simulink model "LUT_kidney_35"  (R2023b)
settings: Solver=FixedStepAuto  StartTime=0  StopTime=10.1  FixedStep=Timegap  RelTol=1e-3
model workspace (MAT data in the model file):
  T1_input = 1.34
(part 1 of 3)
settings Model: Creator=ppxmr2  LastModifiedBy=ppxmr2

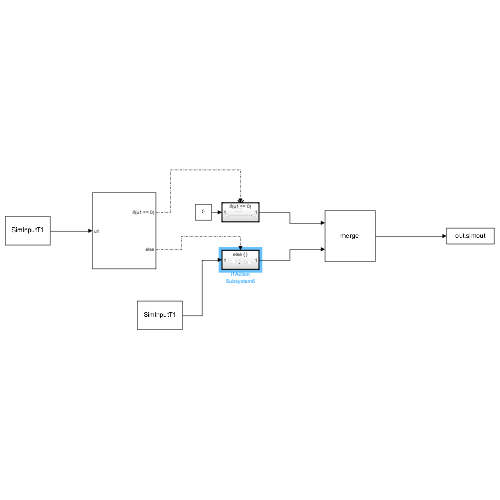
[thumbnail: Simulink's stored preview of the top-level diagram]
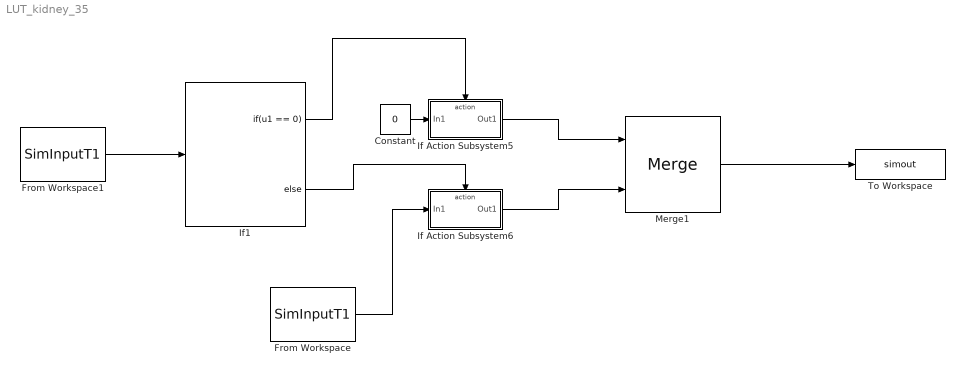
== system LUT_kidney_35 ==
  Constant : Constant  Value=0
  From Workspace : FromWorkspace  VariableName=SimInputT1  Interpolate=off  OutputAfterFinalValue=Setting to zero
  From Workspace1 : FromWorkspace  VariableName=SimInputT1  Interpolate=off  OutputAfterFinalValue=Setting to zero
  If Action Subsystem5 : Subsystem  TreatAsAtomicUnit=on
  If Action Subsystem6 : Subsystem  TreatAsAtomicUnit=on
  If1 : If  IfExpression=u1 == 0
  Merge1 : Merge
  To Workspace : ToWorkspace  VariableName=simout
  wires:
  From Workspace1/1 -> If1/1
  If1/1 -> If Action Subsystem5/Action
  If1/2 -> If Action Subsystem6/Action
  Constant/1 -> If Action Subsystem5/1(In1)
  If Action Subsystem5/1(Out1) -> Merge1/1
  If Action Subsystem6/1(Out1) -> Merge1/2
  Merge1/1 -> To Workspace/1
  From Workspace/1 -> If Action Subsystem6/1(In1)

== system LUT_kidney_35/If Action Subsystem5 ==
  In1 : Inport
  Action Port : ActionPort  ActionPortLabel=if(u1 == 0)
  Out1 : Outport
  wires:
  In1/1 -> Out1/1

== system LUT_kidney_35/If Action Subsystem6 ==
  In1 : Inport
  Action Port : ActionPort  ActionPortLabel=else
  From Workspace1 : FromWorkspace  VariableName=SimInputHR  Interpolate=off  OutputAfterFinalValue=Setting to zero
  If : If  IfExpression=u1 >= 1.495  ElseIfExpressions=u1 >= 0.995
  If Action Subsystem1 : Subsystem  TreatAsAtomicUnit=on
  If Action Subsystem2 : Subsystem  TreatAsAtomicUnit=on
  If Action Subsystem3 : Subsystem  TreatAsAtomicUnit=on
  Merge : Merge  Inputs=3
  Out1 : Outport
  wires:
  Merge/1 -> Out1/1
  From Workspace1/1 -> If/1
  If Action Subsystem1/1(Out1) -> Merge/2
  If Action Subsystem3/1(Out1) -> Merge/3
  In1/1 -> If Action Subsystem2/1(In1), If Action Subsystem1/1(In1), If Action Subsystem3/1(In1)
  If/1 -> If Action Subsystem2/Action
  If/2 -> If Action Subsystem1/Action
  If/3 -> If Action Subsystem3/Action
  If Action Subsystem2/1(Out1) -> Merge/1

== system LUT_kidney_35/If Action Subsystem6/If Action Subsystem1 ==
  In1 : Inport
  Action Port : ActionPort  ActionPortLabel=elseif(u1 >= 0.995)
  From Workspace2 : FromWorkspace  VariableName=SimInputHR  Interpolate=off  OutputAfterFinalValue=Setting to zero
  If Action Subsystem5 : Subsystem  TreatAsAtomicUnit=on
  If Action Subsystem6 : Subsystem  TreatAsAtomicUnit=on
  If Action Subsystem7 : Subsystem  TreatAsAtomicUnit=on
  If Action Subsystem8 : Subsystem  TreatAsAtomicUnit=on
  If Action Subsystem9 : Subsystem  TreatAsAtomicUnit=on
  If1 : If  IfExpression=u1 >= 1.395  ElseIfExpressions=u1 >= 1.295, u1 >= 1.195, u1 >= 1.095
  Merge1 : Merge  Inputs=5
  Out1 : Outport
  wires:
  In1/1 -> If Action Subsystem7/1(In2), If Action Subsystem8/1(In1), If Action Subsystem9/1(In1), If Action Subsystem5/1(In1), If Action Subsystem6/1(In1)
  From Workspace2/1 -> If1/1
  If Action Subsystem9/1(Out1) -> Merge1/1
  If Action Subsystem6/1(Out1) -> Merge1/5
  If Action Subsystem8/1(Out1) -> Merge1/2
  If Action Subsystem5/1(Out1) -> Merge1/4
  If1/4 -> If Action Subsystem5/Action
  If1/2 -> If Action Subsystem8/Action
  If1/3 -> If Action Subsystem7/Action
  If Action Subsystem7/1(Out2) -> Merge1/3
  If1/5 -> If Action Subsystem6/Action
  If1/1 -> If Action Subsystem9/Action
  Merge1/1 -> Out1/1

== system LUT_kidney_35/If Action Subsystem6/If Action Subsystem2 ==
  In1 : Inport
  Action Port : ActionPort  ActionPortLabel=if(u1 >= 1.495)
  From Workspace2 : FromWorkspace  VariableName=SimInputHR  Interpolate=off  OutputAfterFinalValue=Setting to zero
  If Action Subsystem5 : Subsystem  TreatAsAtomicUnit=on
  If Action Subsystem6 : Subsystem  TreatAsAtomicUnit=on
  If Action Subsystem7 : Subsystem  TreatAsAtomicUnit=on
  If Action Subsystem8 : Subsystem  TreatAsAtomicUnit=on
  If Action Subsystem9 : Subsystem  TreatAsAtomicUnit=on
  If1 : If  IfExpression=u1 >= 1.895  ElseIfExpressions=u1 >= 1.795, u1 >= 1.695, u1 >= 1.595
  Merge1 : Merge  Inputs=5
  Out1 : Outport
  wires:
  In1/1 -> If Action Subsystem9/1(In1), If Action Subsystem8/1(In1), If Action Subsystem7/1(In1), If Action Subsystem5/1(In1), If Action Subsystem6/1(In1)
  From Workspace2/1 -> If1/1
  If Action Subsystem9/1(Out1) -> Merge1/1
  If1/4 -> If Action Subsystem5/Action
  If1/2 -> If Action Subsystem8/Action
  If1/3 -> If Action Subsystem7/Action
  If1/5 -> If Action Subsystem6/Action
  If1/1 -> If Action Subsystem9/Action
  Merge1/1 -> Out1/1
  If Action Subsystem8/1(Out1) -> Merge1/2
  If Action Subsystem7/1(Out1) -> Merge1/3
  If Action Subsystem6/1(Out1) -> Merge1/5
  If Action Subsystem5/1(Out1) -> Merge1/4

== system LUT_kidney_35/If Action Subsystem6/If Action Subsystem3 ==
  In1 : Inport
  Action Port : ActionPort  ActionPortLabel=else
  From Workspace2 : FromWorkspace  VariableName=SimInputHR  Interpolate=off  OutputAfterFinalValue=Setting to zero
  If Action Subsystem5 : Subsystem  TreatAsAtomicUnit=on
  If Action Subsystem6 : Subsystem  TreatAsAtomicUnit=on
  If Action Subsystem7 : Subsystem  TreatAsAtomicUnit=on
  If Action Subsystem8 : Subsystem  TreatAsAtomicUnit=on
  If Action Subsystem9 : Subsystem  TreatAsAtomicUnit=on
  If1 : If  IfExpression=u1 >= 0.895  ElseIfExpressions=u1 >= 0.795, u1 >= 0.695, u1 >= 0595
  Merge1 : Merge  Inputs=5
  Out1 : Outport
  wires:
  In1/1 -> If Action Subsystem8/1(In1), If Action Subsystem9/1(In2), If Action Subsystem7/1(In1), If Action Subsystem5/1(In1), If Action Subsystem6/1(In1)
  From Workspace2/1 -> If1/1
  If Action Subsystem9/1(Out2) -> Merge1/1
  If Action Subsystem6/1(Out1) -> Merge1/5
  If Action Subsystem8/1(Out1) -> Merge1/2
  If Action Subsystem5/1(Out1) -> Merge1/4
  If1/4 -> If Action Subsystem5/Action
  If1/2 -> If Action Subsystem8/Action
  If1/3 -> If Action Subsystem7/Action
  If Action Subsystem7/1(Out1) -> Merge1/3
  If1/5 -> If Action Subsystem6/Action
  If1/1 -> If Action Subsystem9/Action
  Merge1/1 -> Out1/1

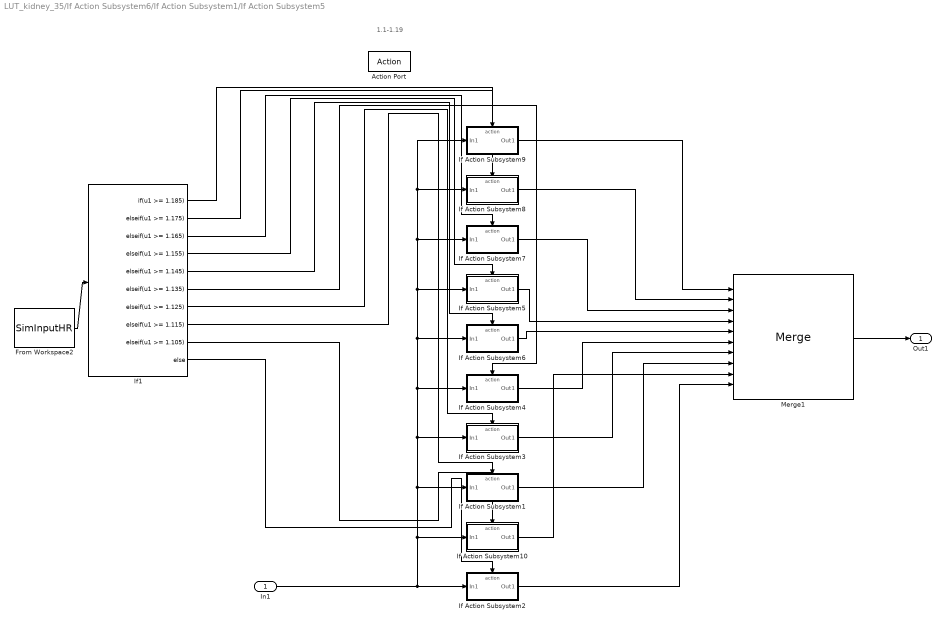
== system LUT_kidney_35/If Action Subsystem6/If Action Subsystem1/If Action Subsystem5 ==
  note: 1.1-1.19
  In1 : Inport
  Action Port : ActionPort  ActionPortLabel=elseif( u1 >= 1.095)
  From Workspace2 : FromWorkspace  VariableName=SimInputHR  Interpolate=off  OutputAfterFinalValue=Setting to zero
  If Action Subsystem1 : Subsystem  TreatAsAtomicUnit=on
  If Action Subsystem10 : Subsystem  TreatAsAtomicUnit=on
  If Action Subsystem2 : Subsystem  TreatAsAtomicUnit=on
  If Action Subsystem3 : Subsystem  TreatAsAtomicUnit=on
  If Action Subsystem4 : Subsystem  TreatAsAtomicUnit=on
  If Action Subsystem5 : Subsystem  TreatAsAtomicUnit=on
  If Action Subsystem6 : Subsystem  TreatAsAtomicUnit=on
  If Action Subsystem7 : Subsystem  TreatAsAtomicUnit=on
  If Action Subsystem8 : Subsystem  TreatAsAtomicUnit=on
  If Action Subsystem9 : Subsystem  TreatAsAtomicUnit=on
  If1 : If  IfExpression=u1 >= 1.185  ElseIfExpressions=u1 >= 1.175, u1 >= 1.165, u1 >= 1.155, u1 >= 1.145, u1 >= 1.135, u1 >= 1.125, u1 >= 1.115, u1 >= 1.105
  Merge1 : Merge  Inputs=10
  Out1 : Outport
  wires:
  If1/10 -> If Action Subsystem2/Action
  If Action Subsystem4/1(Out1) -> Merge1/6
  From Workspace2/1 -> If1/1
  If Action Subsystem6/1(Out1) -> Merge1/5
  Merge1/1 -> Out1/1
  If1/8 -> If Action Subsystem1/Action
  If Action Subsystem3/1(Out1) -> Merge1/7
  In1/1 -> If Action Subsystem1/1(In1), If Action Subsystem3/1(In1), If Action Subsystem4/1(In1), If Action Subsystem7/1(In1), If Action Subsystem8/1(In1), If Action Subsystem9/1(In1), If Action Subsystem5/1(In1), If Action Subsystem6/1(In1), If Action Subsystem10/1(In1), If Action Subsystem2/1(In1)
  If1/6 -> If Action Subsystem4/Action
  If Action Subsystem1/1(Out1) -> Merge1/8
  If1/4 -> If Action Subsystem5/Action
  If Action Subsystem8/1(Out1) -> Merge1/2
  If1/5 -> If Action Subsystem6/Action
  If Action Subsystem7/1(Out1) -> Merge1/3
  If1/3 -> If Action Subsystem7/Action
  If1/7 -> If Action Subsystem3/Action
  If Action Subsystem5/1(Out1) -> Merge1/4
  If Action Subsystem2/1(Out1) -> Merge1/10
  If1/2 -> If Action Subsystem8/Action
  If1/1 -> If Action Subsystem9/Action
  If Action Subsystem9/1(Out1) -> Merge1/1
  If1/9 -> If Action Subsystem10/Action
  If Action Subsystem10/1(Out1) -> Merge1/9

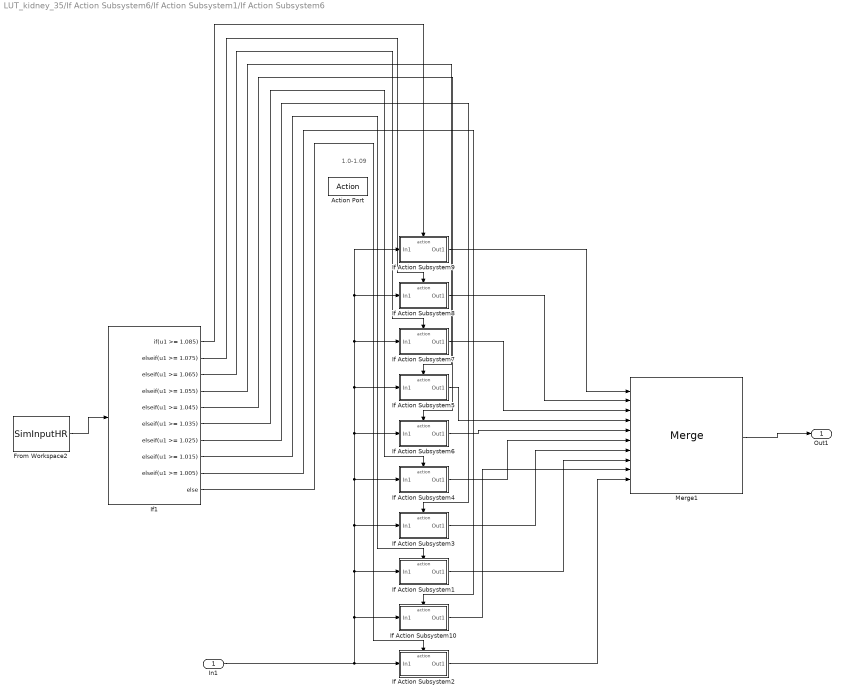
== system LUT_kidney_35/If Action Subsystem6/If Action Subsystem1/If Action Subsystem6 ==
  note: 1.0-1.09
  In1 : Inport
  Action Port : ActionPort  ActionPortLabel=else
  From Workspace2 : FromWorkspace  VariableName=SimInputHR  Interpolate=off  OutputAfterFinalValue=Setting to zero
  If Action Subsystem1 : Subsystem  TreatAsAtomicUnit=on
  If Action Subsystem10 : Subsystem  TreatAsAtomicUnit=on
  If Action Subsystem2 : Subsystem  TreatAsAtomicUnit=on
  If Action Subsystem3 : Subsystem  TreatAsAtomicUnit=on
  If Action Subsystem4 : Subsystem  TreatAsAtomicUnit=on
  If Action Subsystem5 : Subsystem  TreatAsAtomicUnit=on
  If Action Subsystem6 : Subsystem  TreatAsAtomicUnit=on
  If Action Subsystem7 : Subsystem  TreatAsAtomicUnit=on
  If Action Subsystem8 : Subsystem  TreatAsAtomicUnit=on
  If Action Subsystem9 : Subsystem  TreatAsAtomicUnit=on
  If1 : If  IfExpression=u1 >= 1.085  ElseIfExpressions=u1 >= 1.075, u1 >= 1.065, u1 >= 1.055, u1 >= 1.045, u1 >= 1.035, u1 >= 1.025, u1 >= 1.015, u1 >= 1.005
  Merge1 : Merge  Inputs=10
  Out1 : Outport
  wires:
  If1/10 -> If Action Subsystem2/Action
  If Action Subsystem4/1(Out1) -> Merge1/6
  From Workspace2/1 -> If1/1
  If Action Subsystem6/1(Out1) -> Merge1/5
  Merge1/1 -> Out1/1
  If1/8 -> If Action Subsystem1/Action
  If Action Subsystem3/1(Out1) -> Merge1/7
  In1/1 -> If Action Subsystem1/1(In1), If Action Subsystem3/1(In1), If Action Subsystem4/1(In1), If Action Subsystem7/1(In1), If Action Subsystem8/1(In1), If Action Subsystem9/1(In1), If Action Subsystem5/1(In1), If Action Subsystem6/1(In1), If Action Subsystem10/1(In1), If Action Subsystem2/1(In1)
  If1/6 -> If Action Subsystem4/Action
  If Action Subsystem1/1(Out1) -> Merge1/8
  If1/4 -> If Action Subsystem5/Action
  If Action Subsystem8/1(Out1) -> Merge1/2
  If1/5 -> If Action Subsystem6/Action
  If Action Subsystem7/1(Out1) -> Merge1/3
  If1/3 -> If Action Subsystem7/Action
  If1/7 -> If Action Subsystem3/Action
  If Action Subsystem5/1(Out1) -> Merge1/4
  If Action Subsystem2/1(Out1) -> Merge1/10
  If1/2 -> If Action Subsystem8/Action
  If1/1 -> If Action Subsystem9/Action
  If Action Subsystem9/1(Out1) -> Merge1/1
  If1/9 -> If Action Subsystem10/Action
  If Action Subsystem10/1(Out1) -> Merge1/9

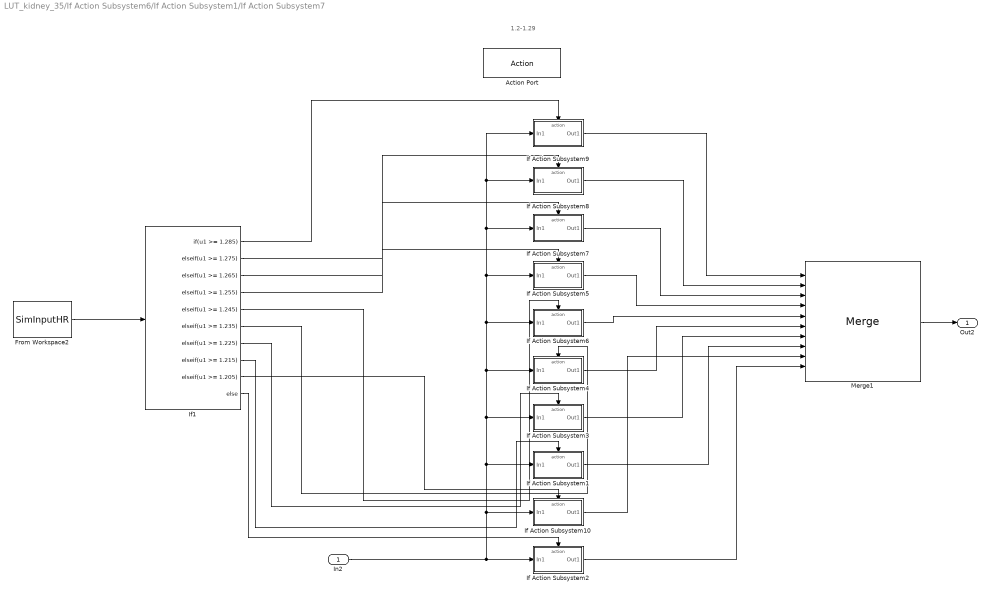
== system LUT_kidney_35/If Action Subsystem6/If Action Subsystem1/If Action Subsystem7 ==
  note: 1.2-1.29
  In2 : Inport
  Action Port : ActionPort  ActionPortLabel=elseif( u1 >= 1.195)
  From Workspace2 : FromWorkspace  VariableName=SimInputHR  Interpolate=off  OutputAfterFinalValue=Setting to zero
  If Action Subsystem1 : Subsystem  TreatAsAtomicUnit=on
  If Action Subsystem10 : Subsystem  TreatAsAtomicUnit=on
  If Action Subsystem2 : Subsystem  TreatAsAtomicUnit=on
  If Action Subsystem3 : Subsystem  TreatAsAtomicUnit=on
  If Action Subsystem4 : Subsystem  TreatAsAtomicUnit=on
  If Action Subsystem5 : Subsystem  TreatAsAtomicUnit=on
  If Action Subsystem6 : Subsystem  TreatAsAtomicUnit=on
  If Action Subsystem7 : Subsystem  TreatAsAtomicUnit=on
  If Action Subsystem8 : Subsystem  TreatAsAtomicUnit=on
  If Action Subsystem9 : Subsystem  TreatAsAtomicUnit=on
  If1 : If  IfExpression=u1 >= 1.285  ElseIfExpressions=u1 >= 1.275, u1 >= 1.265, u1 >= 1.255, u1 >= 1.245, u1 >= 1.235, u1 >= 1.225, u1 >= 1.215, u1 >= 1.205
  Merge1 : Merge  Inputs=10
  Out2 : Outport
  wires:
  If1/10 -> If Action Subsystem2/Action
  If Action Subsystem4/1(Out1) -> Merge1/6
  From Workspace2/1 -> If1/1
  If Action Subsystem6/1(Out1) -> Merge1/5
  Merge1/1 -> Out2/1
  If1/8 -> If Action Subsystem1/Action
  If Action Subsystem3/1(Out1) -> Merge1/7
  In2/1 -> If Action Subsystem1/1(In1), If Action Subsystem3/1(In1), If Action Subsystem4/1(In1), If Action Subsystem7/1(In1), If Action Subsystem8/1(In1), If Action Subsystem9/1(In1), If Action Subsystem5/1(In1), If Action Subsystem6/1(In1), If Action Subsystem10/1(In1), If Action Subsystem2/1(In1)
  If1/6 -> If Action Subsystem4/Action
  If Action Subsystem1/1(Out1) -> Merge1/8
  If1/4 -> If Action Subsystem5/Action
  If Action Subsystem8/1(Out1) -> Merge1/2
  If1/5 -> If Action Subsystem6/Action
  If Action Subsystem7/1(Out1) -> Merge1/3
  If1/3 -> If Action Subsystem7/Action
  If1/7 -> If Action Subsystem3/Action
  If Action Subsystem5/1(Out1) -> Merge1/4
  If Action Subsystem2/1(Out1) -> Merge1/10
  If1/2 -> If Action Subsystem8/Action
  If1/1 -> If Action Subsystem9/Action
  If Action Subsystem9/1(Out1) -> Merge1/1
  If Action Subsystem10/1(Out1) -> Merge1/9
  If1/9 -> If Action Subsystem10/Action

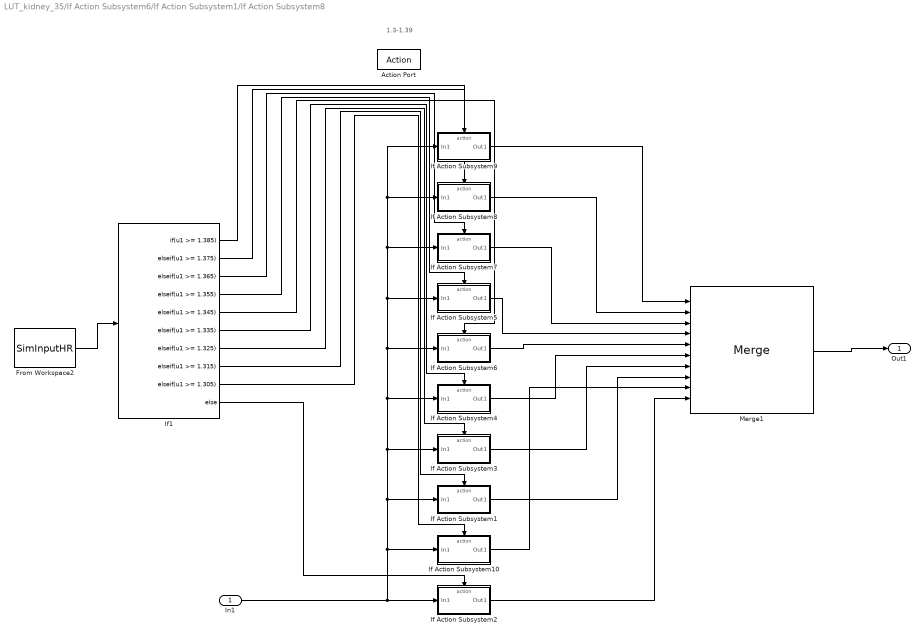
== system LUT_kidney_35/If Action Subsystem6/If Action Subsystem1/If Action Subsystem8 ==
  note: 1.3-1.39
  In1 : Inport
  Action Port : ActionPort  ActionPortLabel=elseif(u1 >= 1.295)
  From Workspace2 : FromWorkspace  VariableName=SimInputHR  Interpolate=off  OutputAfterFinalValue=Setting to zero
  If Action Subsystem1 : Subsystem  TreatAsAtomicUnit=on
  If Action Subsystem10 : Subsystem  TreatAsAtomicUnit=on
  If Action Subsystem2 : Subsystem  TreatAsAtomicUnit=on
  If Action Subsystem3 : Subsystem  TreatAsAtomicUnit=on
  If Action Subsystem4 : Subsystem  TreatAsAtomicUnit=on
  If Action Subsystem5 : Subsystem  TreatAsAtomicUnit=on
  If Action Subsystem6 : Subsystem  TreatAsAtomicUnit=on
  If Action Subsystem7 : Subsystem  TreatAsAtomicUnit=on
  If Action Subsystem8 : Subsystem  TreatAsAtomicUnit=on
  If Action Subsystem9 : Subsystem  TreatAsAtomicUnit=on
  If1 : If  IfExpression=u1 >= 1.385  ElseIfExpressions=u1 >= 1.375, u1 >= 1.365, u1 >= 1.355, u1 >= 1.345, u1 >= 1.335, u1 >= 1.325, u1 >= 1.315, u1 >= 1.305
  Merge1 : Merge  Inputs=10
  Out1 : Outport
  wires:
  If1/10 -> If Action Subsystem2/Action
  If Action Subsystem4/1(Out1) -> Merge1/6
  From Workspace2/1 -> If1/1
  If Action Subsystem6/1(Out1) -> Merge1/5
  Merge1/1 -> Out1/1
  If1/8 -> If Action Subsystem1/Action
  If Action Subsystem3/1(Out1) -> Merge1/7
  In1/1 -> If Action Subsystem1/1(In1), If Action Subsystem3/1(In1), If Action Subsystem4/1(In1), If Action Subsystem7/1(In1), If Action Subsystem8/1(In1), If Action Subsystem9/1(In1), If Action Subsystem5/1(In1), If Action Subsystem6/1(In1), If Action Subsystem10/1(In1), If Action Subsystem2/1(In1)
  If1/6 -> If Action Subsystem4/Action
  If Action Subsystem1/1(Out1) -> Merge1/8
  If1/4 -> If Action Subsystem5/Action
  If Action Subsystem8/1(Out1) -> Merge1/2
  If1/5 -> If Action Subsystem6/Action
  If Action Subsystem7/1(Out1) -> Merge1/3
  If1/3 -> If Action Subsystem7/Action
  If1/7 -> If Action Subsystem3/Action
  If Action Subsystem5/1(Out1) -> Merge1/4
  If Action Subsystem2/1(Out1) -> Merge1/10
  If1/2 -> If Action Subsystem8/Action
  If1/1 -> If Action Subsystem9/Action
  If Action Subsystem9/1(Out1) -> Merge1/1
  If1/9 -> If Action Subsystem10/Action
  If Action Subsystem10/1(Out1) -> Merge1/9

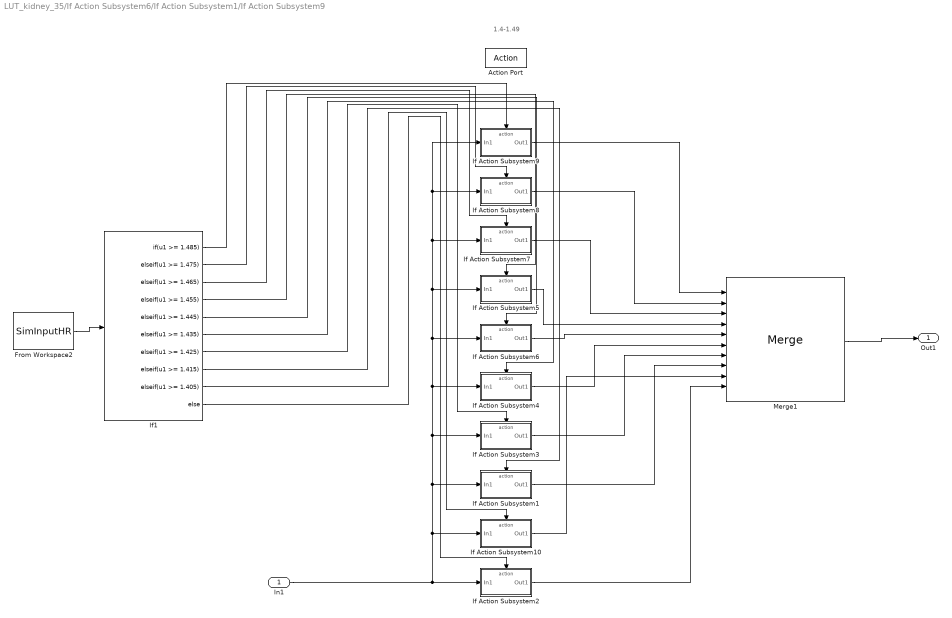
== system LUT_kidney_35/If Action Subsystem6/If Action Subsystem1/If Action Subsystem9 ==
  note: 1.4-1.49
  In1 : Inport
  Action Port : ActionPort  ActionPortLabel=if(u1 >= 1.395)
  From Workspace2 : FromWorkspace  VariableName=SimInputHR  Interpolate=off  OutputAfterFinalValue=Setting to zero
  If Action Subsystem1 : Subsystem  TreatAsAtomicUnit=on
  If Action Subsystem10 : Subsystem  TreatAsAtomicUnit=on
  If Action Subsystem2 : Subsystem  TreatAsAtomicUnit=on
  If Action Subsystem3 : Subsystem  TreatAsAtomicUnit=on
  If Action Subsystem4 : Subsystem  TreatAsAtomicUnit=on
  If Action Subsystem5 : Subsystem  TreatAsAtomicUnit=on
  If Action Subsystem6 : Subsystem  TreatAsAtomicUnit=on
  If Action Subsystem7 : Subsystem  TreatAsAtomicUnit=on
  If Action Subsystem8 : Subsystem  TreatAsAtomicUnit=on
  If Action Subsystem9 : Subsystem  TreatAsAtomicUnit=on
  If1 : If  IfExpression=u1 >= 1.485  ElseIfExpressions=u1 >= 1.475, u1 >= 1.465, u1 >= 1.455, u1 >= 1.445, u1 >= 1.435, u1 >= 1.425, u1 >= 1.415, u1 >= 1.405
  Merge1 : Merge  Inputs=10
  Out1 : Outport
  wires:
  If1/10 -> If Action Subsystem2/Action
  If Action Subsystem4/1(Out1) -> Merge1/6
  From Workspace2/1 -> If1/1
  If Action Subsystem6/1(Out1) -> Merge1/5
  Merge1/1 -> Out1/1
  If1/8 -> If Action Subsystem1/Action
  If Action Subsystem3/1(Out1) -> Merge1/7
  In1/1 -> If Action Subsystem10/1(In1), If Action Subsystem1/1(In1), If Action Subsystem3/1(In1), If Action Subsystem4/1(In1), If Action Subsystem7/1(In1), If Action Subsystem8/1(In1), If Action Subsystem9/1(In1), If Action Subsystem5/1(In1), If Action Subsystem6/1(In1), If Action Subsystem2/1(In1)
  If1/6 -> If Action Subsystem4/Action
  If Action Subsystem1/1(Out1) -> Merge1/8
  If1/4 -> If Action Subsystem5/Action
  If Action Subsystem8/1(Out1) -> Merge1/2
  If1/5 -> If Action Subsystem6/Action
  If Action Subsystem7/1(Out1) -> Merge1/3
  If1/3 -> If Action Subsystem7/Action
  If1/7 -> If Action Subsystem3/Action
  If Action Subsystem5/1(Out1) -> Merge1/4
  If Action Subsystem2/1(Out1) -> Merge1/10
  If1/2 -> If Action Subsystem8/Action
  If1/1 -> If Action Subsystem9/Action
  If Action Subsystem9/1(Out1) -> Merge1/1
  If1/9 -> If Action Subsystem10/Action
  If Action Subsystem10/1(Out1) -> Merge1/9

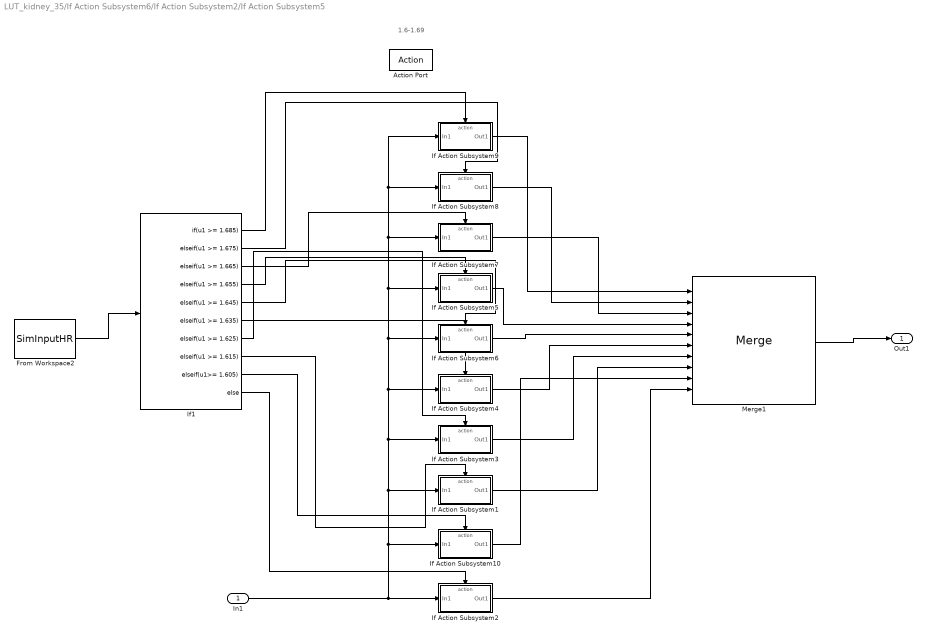
== system LUT_kidney_35/If Action Subsystem6/If Action Subsystem2/If Action Subsystem5 ==
  note: 1.6-1.69
  In1 : Inport
  Action Port : ActionPort  ActionPortLabel=elseif( u1 >= 1.595)
  From Workspace2 : FromWorkspace  VariableName=SimInputHR  Interpolate=off  OutputAfterFinalValue=Setting to zero
  If Action Subsystem1 : Subsystem  TreatAsAtomicUnit=on
  If Action Subsystem10 : Subsystem  TreatAsAtomicUnit=on
  If Action Subsystem2 : Subsystem  TreatAsAtomicUnit=on
  If Action Subsystem3 : Subsystem  TreatAsAtomicUnit=on
  If Action Subsystem4 : Subsystem  TreatAsAtomicUnit=on
  If Action Subsystem5 : Subsystem  TreatAsAtomicUnit=on
  If Action Subsystem6 : Subsystem  TreatAsAtomicUnit=on
  If Action Subsystem7 : Subsystem  TreatAsAtomicUnit=on
  If Action Subsystem8 : Subsystem  TreatAsAtomicUnit=on
  If Action Subsystem9 : Subsystem  TreatAsAtomicUnit=on
  If1 : If  IfExpression=u1 >= 1.685  ElseIfExpressions=u1 >= 1.675, u1 >= 1.665, u1 >= 1.655, u1 >= 1.645, u1 >= 1.635, u1 >= 1.625, u1 >= 1.615, u1>= 1.605
  Merge1 : Merge  Inputs=10
  Out1 : Outport
  wires:
  If1/2 -> If Action Subsystem8/Action
  If Action Subsystem5/1(Out1) -> Merge1/4
  If1/3 -> If Action Subsystem7/Action
  If Action Subsystem9/1(Out1) -> Merge1/1
  If1/7 -> If Action Subsystem3/Action
  If1/5 -> If Action Subsystem6/Action
  If1/1 -> If Action Subsystem9/Action
  If Action Subsystem4/1(Out1) -> Merge1/6
  If1/10 -> If Action Subsystem2/Action
  If Action Subsystem8/1(Out1) -> Merge1/2
  If1/4 -> If Action Subsystem5/Action
  In1/1 -> If Action Subsystem10/1(In1), If Action Subsystem1/1(In1), If Action Subsystem3/1(In1), If Action Subsystem4/1(In1), If Action Subsystem7/1(In1), If Action Subsystem8/1(In1), If Action Subsystem9/1(In1), If Action Subsystem5/1(In1), If Action Subsystem6/1(In1), If Action Subsystem2/1(In1)
  If Action Subsystem1/1(Out1) -> Merge1/8
  If Action Subsystem2/1(Out1) -> Merge1/10
  If1/8 -> If Action Subsystem1/Action
  If Action Subsystem3/1(Out1) -> Merge1/7
  If1/6 -> If Action Subsystem4/Action
  From Workspace2/1 -> If1/1
  Merge1/1 -> Out1/1
  If Action Subsystem6/1(Out1) -> Merge1/5
  If Action Subsystem7/1(Out1) -> Merge1/3
  If1/9 -> If Action Subsystem10/Action
  If Action Subsystem10/1(Out1) -> Merge1/9

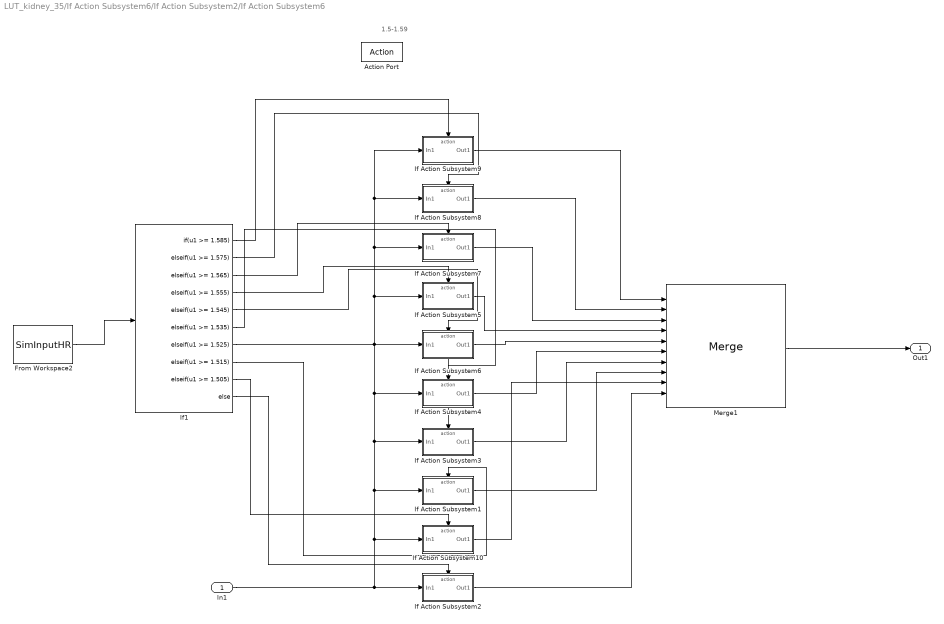
== system LUT_kidney_35/If Action Subsystem6/If Action Subsystem2/If Action Subsystem6 ==
  note: 1.5-1.59
  In1 : Inport
  Action Port : ActionPort  ActionPortLabel=else
  From Workspace2 : FromWorkspace  VariableName=SimInputHR  Interpolate=off  OutputAfterFinalValue=Setting to zero
  If Action Subsystem1 : Subsystem  TreatAsAtomicUnit=on
  If Action Subsystem10 : Subsystem  TreatAsAtomicUnit=on
  If Action Subsystem2 : Subsystem  TreatAsAtomicUnit=on
  If Action Subsystem3 : Subsystem  TreatAsAtomicUnit=on
  If Action Subsystem4 : Subsystem  TreatAsAtomicUnit=on
  If Action Subsystem5 : Subsystem  TreatAsAtomicUnit=on
  If Action Subsystem6 : Subsystem  TreatAsAtomicUnit=on
  If Action Subsystem7 : Subsystem  TreatAsAtomicUnit=on
  If Action Subsystem8 : Subsystem  TreatAsAtomicUnit=on
  If Action Subsystem9 : Subsystem  TreatAsAtomicUnit=on
  If1 : If  IfExpression=u1 >= 1.585  ElseIfExpressions=u1 >= 1.575, u1 >= 1.565, u1 >= 1.555, u1 >= 1.545, u1 >= 1.535, u1 >= 1.525, u1 >= 1.515, u1 >= 1.505
  Merge1 : Merge  Inputs=10
  Out1 : Outport
  wires:
  If1/2 -> If Action Subsystem8/Action
  If Action Subsystem5/1(Out1) -> Merge1/4
  If1/3 -> If Action Subsystem7/Action
  If Action Subsystem9/1(Out1) -> Merge1/1
  If1/7 -> If Action Subsystem3/Action
  If1/5 -> If Action Subsystem6/Action
  If1/1 -> If Action Subsystem9/Action
  If Action Subsystem4/1(Out1) -> Merge1/6
  If1/10 -> If Action Subsystem2/Action
  If Action Subsystem8/1(Out1) -> Merge1/2
  If1/4 -> If Action Subsystem5/Action
  In1/1 -> If Action Subsystem10/1(In1), If Action Subsystem1/1(In1), If Action Subsystem3/1(In1), If Action Subsystem4/1(In1), If Action Subsystem7/1(In1), If Action Subsystem8/1(In1), If Action Subsystem9/1(In1), If Action Subsystem5/1(In1), If Action Subsystem6/1(In1), If Action Subsystem2/1(In1)
  If Action Subsystem1/1(Out1) -> Merge1/8
  If Action Subsystem2/1(Out1) -> Merge1/10
  If1/8 -> If Action Subsystem1/Action
  If Action Subsystem3/1(Out1) -> Merge1/7
  If1/6 -> If Action Subsystem4/Action
  From Workspace2/1 -> If1/1
  Merge1/1 -> Out1/1
  If Action Subsystem6/1(Out1) -> Merge1/5
  If Action Subsystem7/1(Out1) -> Merge1/3
  If1/9 -> If Action Subsystem10/Action
  If Action Subsystem10/1(Out1) -> Merge1/9

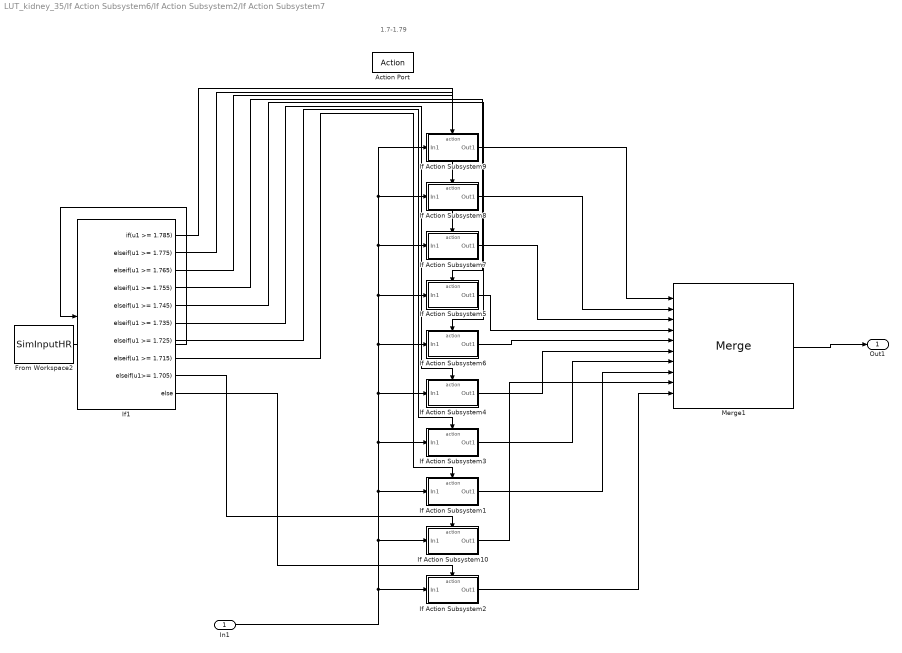
== system LUT_kidney_35/If Action Subsystem6/If Action Subsystem2/If Action Subsystem7 ==
  note: 1.7-1.79
  In1 : Inport
  Action Port : ActionPort  ActionPortLabel=elseif( u1 >= 1.695)
  From Workspace2 : FromWorkspace  VariableName=SimInputHR  Interpolate=off  OutputAfterFinalValue=Setting to zero
  If Action Subsystem1 : Subsystem  TreatAsAtomicUnit=on
  If Action Subsystem10 : Subsystem  TreatAsAtomicUnit=on
  If Action Subsystem2 : Subsystem  TreatAsAtomicUnit=on
  If Action Subsystem3 : Subsystem  TreatAsAtomicUnit=on
  If Action Subsystem4 : Subsystem  TreatAsAtomicUnit=on
  If Action Subsystem5 : Subsystem  TreatAsAtomicUnit=on
  If Action Subsystem6 : Subsystem  TreatAsAtomicUnit=on
  If Action Subsystem7 : Subsystem  TreatAsAtomicUnit=on
  If Action Subsystem8 : Subsystem  TreatAsAtomicUnit=on
  If Action Subsystem9 : Subsystem  TreatAsAtomicUnit=on
  If1 : If  IfExpression=u1 >= 1.785  ElseIfExpressions=u1 >= 1.775, u1 >= 1.765, u1 >= 1.755, u1 >= 1.745, u1 >= 1.735, u1 >= 1.725, u1 >= 1.715, u1>= 1.705
  Merge1 : Merge  Inputs=10
  Out1 : Outport
  wires:
  If1/2 -> If Action Subsystem8/Action
  If Action Subsystem5/1(Out1) -> Merge1/4
  If1/3 -> If Action Subsystem7/Action
  If Action Subsystem9/1(Out1) -> Merge1/1
  If1/7 -> If Action Subsystem3/Action
  If1/5 -> If Action Subsystem6/Action
  If1/1 -> If Action Subsystem9/Action
  If Action Subsystem4/1(Out1) -> Merge1/6
  If1/10 -> If Action Subsystem2/Action
  If Action Subsystem8/1(Out1) -> Merge1/2
  If1/4 -> If Action Subsystem5/Action
  In1/1 -> If Action Subsystem10/1(In1), If Action Subsystem1/1(In1), If Action Subsystem3/1(In1), If Action Subsystem4/1(In1), If Action Subsystem7/1(In1), If Action Subsystem8/1(In1), If Action Subsystem9/1(In1), If Action Subsystem5/1(In1), If Action Subsystem6/1(In1), If Action Subsystem2/1(In1)
  If Action Subsystem1/1(Out1) -> Merge1/8
  If Action Subsystem2/1(Out1) -> Merge1/10
  If1/8 -> If Action Subsystem1/Action
  If Action Subsystem3/1(Out1) -> Merge1/7
  If1/6 -> If Action Subsystem4/Action
  From Workspace2/1 -> If1/1
  Merge1/1 -> Out1/1
  If Action Subsystem6/1(Out1) -> Merge1/5
  If Action Subsystem7/1(Out1) -> Merge1/3
  If Action Subsystem10/1(Out1) -> Merge1/9
  If1/9 -> If Action Subsystem10/Action

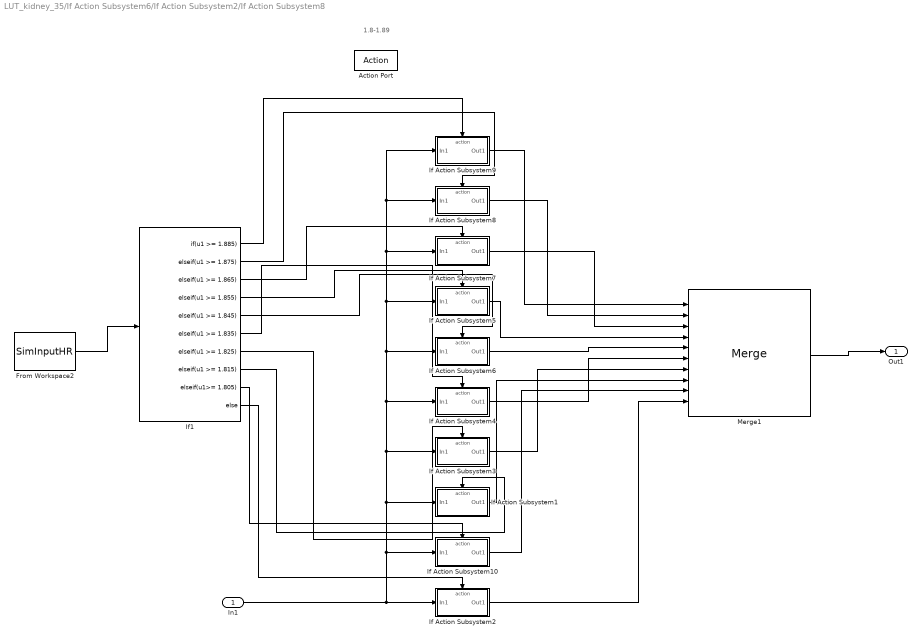
== system LUT_kidney_35/If Action Subsystem6/If Action Subsystem2/If Action Subsystem8 ==
  note: 1.8-1.89
  In1 : Inport
  Action Port : ActionPort  ActionPortLabel=elseif(u1 >= 1.795)
  From Workspace2 : FromWorkspace  VariableName=SimInputHR  Interpolate=off  OutputAfterFinalValue=Setting to zero
  If Action Subsystem1 : Subsystem  TreatAsAtomicUnit=on
  If Action Subsystem10 : Subsystem  TreatAsAtomicUnit=on
  If Action Subsystem2 : Subsystem  TreatAsAtomicUnit=on
  If Action Subsystem3 : Subsystem  TreatAsAtomicUnit=on
  If Action Subsystem4 : Subsystem  TreatAsAtomicUnit=on
  If Action Subsystem5 : Subsystem  TreatAsAtomicUnit=on
  If Action Subsystem6 : Subsystem  TreatAsAtomicUnit=on
  If Action Subsystem7 : Subsystem  TreatAsAtomicUnit=on
  If Action Subsystem8 : Subsystem  TreatAsAtomicUnit=on
  If Action Subsystem9 : Subsystem  TreatAsAtomicUnit=on
  If1 : If  IfExpression=u1 >= 1.885  ElseIfExpressions=u1 >= 1.875, u1 >= 1.865, u1 >= 1.855, u1 >= 1.845, u1 >= 1.835, u1 >= 1.825, u1 >= 1.815, u1>= 1.805
  Merge1 : Merge  Inputs=10
  Out1 : Outport
  wires:
  If1/2 -> If Action Subsystem8/Action
  If Action Subsystem5/1(Out1) -> Merge1/4
  If1/3 -> If Action Subsystem7/Action
  If Action Subsystem9/1(Out1) -> Merge1/1
  If1/7 -> If Action Subsystem3/Action
  If1/5 -> If Action Subsystem6/Action
  If1/1 -> If Action Subsystem9/Action
  If Action Subsystem4/1(Out1) -> Merge1/6
  If1/10 -> If Action Subsystem2/Action
  If Action Subsystem8/1(Out1) -> Merge1/2
  If1/4 -> If Action Subsystem5/Action
  In1/1 -> If Action Subsystem10/1(In1), If Action Subsystem1/1(In1), If Action Subsystem3/1(In1), If Action Subsystem4/1(In1), If Action Subsystem7/1(In1), If Action Subsystem8/1(In1), If Action Subsystem9/1(In1), If Action Subsystem5/1(In1), If Action Subsystem6/1(In1), If Action Subsystem2/1(In1)
  If Action Subsystem1/1(Out1) -> Merge1/8
  If Action Subsystem2/1(Out1) -> Merge1/10
  If1/8 -> If Action Subsystem1/Action
  If Action Subsystem3/1(Out1) -> Merge1/7
  If1/6 -> If Action Subsystem4/Action
  From Workspace2/1 -> If1/1
  Merge1/1 -> Out1/1
  If Action Subsystem6/1(Out1) -> Merge1/5
  If Action Subsystem7/1(Out1) -> Merge1/3
  If1/9 -> If Action Subsystem10/Action
  If Action Subsystem10/1(Out1) -> Merge1/9

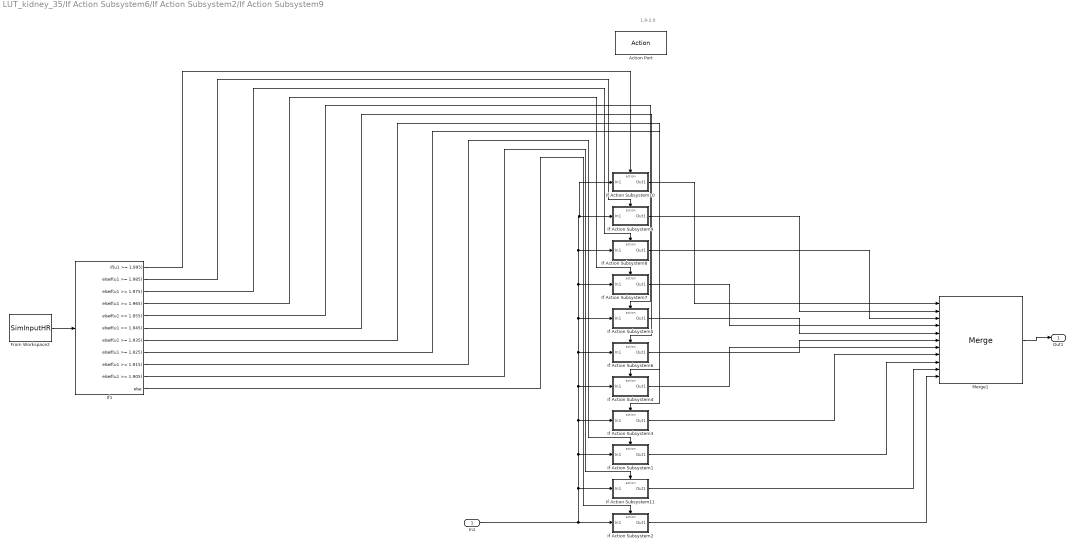
== system LUT_kidney_35/If Action Subsystem6/If Action Subsystem2/If Action Subsystem9 ==
  note: 1.9-2.0
  In1 : Inport
  Action Port : ActionPort  ActionPortLabel=if(u1 >= 1.895)
  From Workspace2 : FromWorkspace  VariableName=SimInputHR  Interpolate=off  OutputAfterFinalValue=Setting to zero
  If Action Subsystem1 : Subsystem  TreatAsAtomicUnit=on
  If Action Subsystem10 : Subsystem  TreatAsAtomicUnit=on
  If Action Subsystem11 : Subsystem  TreatAsAtomicUnit=on
  If Action Subsystem2 : Subsystem  TreatAsAtomicUnit=on
  If Action Subsystem3 : Subsystem  TreatAsAtomicUnit=on
  If Action Subsystem4 : Subsystem  TreatAsAtomicUnit=on
  If Action Subsystem5 : Subsystem  TreatAsAtomicUnit=on
  If Action Subsystem6 : Subsystem  TreatAsAtomicUnit=on
  If Action Subsystem7 : Subsystem  TreatAsAtomicUnit=on
  If Action Subsystem8 : Subsystem  TreatAsAtomicUnit=on
  If Action Subsystem9 : Subsystem  TreatAsAtomicUnit=on
  If1 : If  IfExpression=u1 >= 1.995  ElseIfExpressions=u1 >= 1.985, u1 >= 1.975, u1 >= 1.965, u1 >= 1.955, u1 >= 1.945, u1 >= 1.935, u1 >= 1.925, u1 >= 1.915, u1 >= 1.905
  Merge1 : Merge  Inputs=11
  Out1 : Outport
  wires:
  Merge1/1 -> Out1/1
  From Workspace2/1 -> If1/1
  If1/2 -> If Action Subsystem9/Action
  If1/3 -> If Action Subsystem8/Action
  If1/4 -> If Action Subsystem7/Action
  If1/5 -> If Action Subsystem5/Action
  If1/6 -> If Action Subsystem6/Action
  If1/7 -> If Action Subsystem4/Action
  If1/8 -> If Action Subsystem3/Action
  If1/9 -> If Action Subsystem1/Action
  If1/11 -> If Action Subsystem2/Action
  If Action Subsystem9/1(Out1) -> Merge1/2
  If Action Subsystem8/1(Out1) -> Merge1/3
  If Action Subsystem7/1(Out1) -> Merge1/4
  If Action Subsystem5/1(Out1) -> Merge1/5
  If Action Subsystem6/1(Out1) -> Merge1/6
  If Action Subsystem4/1(Out1) -> Merge1/7
  If Action Subsystem3/1(Out1) -> Merge1/8
  If Action Subsystem2/1(Out1) -> Merge1/11
  If Action Subsystem1/1(Out1) -> Merge1/9
  In1/1 -> If Action Subsystem1/1(In1), If Action Subsystem3/1(In1), If Action Subsystem4/1(In1), If Action Subsystem7/1(In1), If Action Subsystem8/1(In1), If Action Subsystem10/1(In1), If Action Subsystem9/1(In1), If Action Subsystem5/1(In1), If Action Subsystem6/1(In1), If Action Subsystem11/1(In1), If Action Subsystem2/1(In1)
  If1/1 -> If Action Subsystem10/Action
  If Action Subsystem10/1(Out1) -> Merge1/1
  If1/10 -> If Action Subsystem11/Action
  If Action Subsystem11/1(Out1) -> Merge1/10

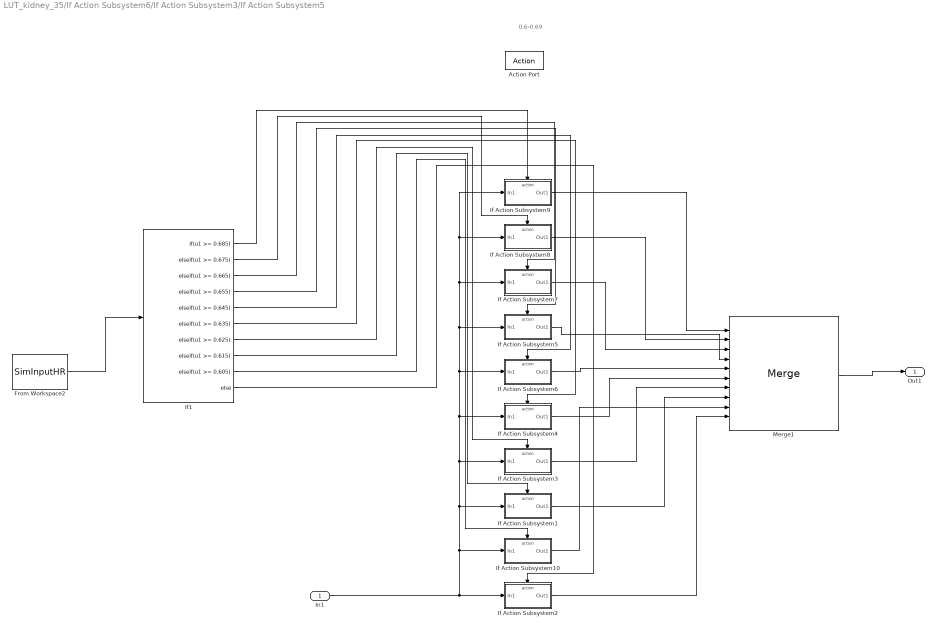
== system LUT_kidney_35/If Action Subsystem6/If Action Subsystem3/If Action Subsystem5 ==
  note: 0.6-0.69
  In1 : Inport
  Action Port : ActionPort  ActionPortLabel=elseif( u1 >= 0595)
  From Workspace2 : FromWorkspace  VariableName=SimInputHR  Interpolate=off  OutputAfterFinalValue=Setting to zero
  If Action Subsystem1 : Subsystem  TreatAsAtomicUnit=on
  If Action Subsystem10 : Subsystem  TreatAsAtomicUnit=on
  If Action Subsystem2 : Subsystem  TreatAsAtomicUnit=on
  If Action Subsystem3 : Subsystem  TreatAsAtomicUnit=on
  If Action Subsystem4 : Subsystem  TreatAsAtomicUnit=on
  If Action Subsystem5 : Subsystem  TreatAsAtomicUnit=on
  If Action Subsystem6 : Subsystem  TreatAsAtomicUnit=on
  If Action Subsystem7 : Subsystem  TreatAsAtomicUnit=on
  If Action Subsystem8 : Subsystem  TreatAsAtomicUnit=on
  If Action Subsystem9 : Subsystem  TreatAsAtomicUnit=on
  If1 : If  IfExpression=u1 >= 0.685  ElseIfExpressions=u1 >= 0.675, u1 >= 0.665, u1 >= 0.655, u1 >= 0.645, u1 >= 0.635, u1 >= 0.625, u1 >= 0.615, u1 >= 0.605
  Merge1 : Merge  Inputs=10
  Out1 : Outport
  wires:
  If1/10 -> If Action Subsystem2/Action
  If Action Subsystem4/1(Out1) -> Merge1/6
  From Workspace2/1 -> If1/1
  If Action Subsystem6/1(Out1) -> Merge1/5
  Merge1/1 -> Out1/1
  If1/8 -> If Action Subsystem1/Action
  If Action Subsystem3/1(Out1) -> Merge1/7
  In1/1 -> If Action Subsystem1/1(In1), If Action Subsystem3/1(In1), If Action Subsystem4/1(In1), If Action Subsystem7/1(In1), If Action Subsystem8/1(In1), If Action Subsystem9/1(In1), If Action Subsystem5/1(In1), If Action Subsystem6/1(In1), If Action Subsystem10/1(In1), If Action Subsystem2/1(In1)
  If1/6 -> If Action Subsystem4/Action
  If Action Subsystem1/1(Out1) -> Merge1/8
  If1/4 -> If Action Subsystem5/Action
  If Action Subsystem8/1(Out1) -> Merge1/2
  If1/5 -> If Action Subsystem6/Action
  If Action Subsystem7/1(Out1) -> Merge1/3
  If1/3 -> If Action Subsystem7/Action
  If1/7 -> If Action Subsystem3/Action
  If Action Subsystem5/1(Out1) -> Merge1/4
  If Action Subsystem2/1(Out1) -> Merge1/10
  If1/2 -> If Action Subsystem8/Action
  If1/1 -> If Action Subsystem9/Action
  If Action Subsystem9/1(Out1) -> Merge1/1
  If Action Subsystem10/1(Out1) -> Merge1/9
  If1/9 -> If Action Subsystem10/Action

== system LUT_kidney_35/If Action Subsystem6/If Action Subsystem3/If Action Subsystem6 ==
  note: 0.5-0.59
  In1 : Inport
  Action Port : ActionPort  ActionPortLabel=else
  From Workspace2 : FromWorkspace  VariableName=SimInputHR  Interpolate=off  OutputAfterFinalValue=Setting to zero
  If Action Subsystem1 : Subsystem  TreatAsAtomicUnit=on
  If Action Subsystem10 : Subsystem  TreatAsAtomicUnit=on
  If Action Subsystem2 : Subsystem  TreatAsAtomicUnit=on
  If Action Subsystem3 : Subsystem  TreatAsAtomicUnit=on
  If Action Subsystem4 : Subsystem  TreatAsAtomicUnit=on
  If Action Subsystem5 : Subsystem  TreatAsAtomicUnit=on
  If Action Subsystem6 : Subsystem  TreatAsAtomicUnit=on
  If Action Subsystem7 : Subsystem  TreatAsAtomicUnit=on
  If Action Subsystem8 : Subsystem  TreatAsAtomicUnit=on
  If Action Subsystem9 : Subsystem  TreatAsAtomicUnit=on
  If1 : If  IfExpression=u1 >= 0.585  ElseIfExpressions=u1 >= 0.575, u1 >= 0.565, u1 >= 0.555, u1 >= 0.545, u1 >= 0.535, u1 >= 0.525, u1 >= 0.515, u1 >= 0.505
  Merge1 : Merge  Inputs=10
  Out1 : Outport
  wires:
  If1/10 -> If Action Subsystem2/Action
  If Action Subsystem4/1(Out1) -> Merge1/6
  From Workspace2/1 -> If1/1
  If Action Subsystem6/1(Out1) -> Merge1/5
  Merge1/1 -> Out1/1
  If1/8 -> If Action Subsystem1/Action
  If Action Subsystem3/1(Out1) -> Merge1/7
  In1/1 -> If Action Subsystem1/1(In1), If Action Subsystem3/1(In1), If Action Subsystem4/1(In1), If Action Subsystem7/1(In1), If Action Subsystem8/1(In1), If Action Subsystem9/1(In1), If Action Subsystem5/1(In1), If Action Subsystem6/1(In1), If Action Subsystem10/1(In1), If Action Subsystem2/1(In1)
  If1/6 -> If Action Subsystem4/Action
  If Action Subsystem1/1(Out1) -> Merge1/8
  If1/4 -> If Action Subsystem5/Action
  If Action Subsystem8/1(Out1) -> Merge1/2
  If1/5 -> If Action Subsystem6/Action
  If Action Subsystem7/1(Out1) -> Merge1/3
  If1/3 -> If Action Subsystem7/Action
  If1/7 -> If Action Subsystem3/Action
  If Action Subsystem5/1(Out1) -> Merge1/4
  If Action Subsystem2/1(Out1) -> Merge1/10
  If1/2 -> If Action Subsystem8/Action
  If1/1 -> If Action Subsystem9/Action
  If Action Subsystem9/1(Out1) -> Merge1/1
  If Action Subsystem10/1(Out1) -> Merge1/9
  If1/9 -> If Action Subsystem10/Action

== system LUT_kidney_35/If Action Subsystem6/If Action Subsystem3/If Action Subsystem7 ==
  note: 0.7-0.79
  In1 : Inport
  Action Port : ActionPort  ActionPortLabel=elseif( u1 >= 0.695)
  From Workspace2 : FromWorkspace  VariableName=SimInputHR  Interpolate=off  OutputAfterFinalValue=Setting to zero
  If Action Subsystem1 : Subsystem  TreatAsAtomicUnit=on
  If Action Subsystem10 : Subsystem  TreatAsAtomicUnit=on
  If Action Subsystem2 : Subsystem  TreatAsAtomicUnit=on
  If Action Subsystem3 : Subsystem  TreatAsAtomicUnit=on
  If Action Subsystem4 : Subsystem  TreatAsAtomicUnit=on
  If Action Subsystem5 : Subsystem  TreatAsAtomicUnit=on
  If Action Subsystem6 : Subsystem  TreatAsAtomicUnit=on
  If Action Subsystem7 : Subsystem  TreatAsAtomicUnit=on
  If Action Subsystem8 : Subsystem  TreatAsAtomicUnit=on
  If Action Subsystem9 : Subsystem  TreatAsAtomicUnit=on
  If1 : If  IfExpression=u1 >= 0.785  ElseIfExpressions=u1 >= 0.775, u1 >= 0.765, u1 >= 0.755, u1 >= 0.745, u1 >= 0.735, u1 >= 0.725, u1 >= 0.715, u1 >= 0.705
  Merge1 : Merge  Inputs=10
  Out1 : Outport
  wires:
  If1/10 -> If Action Subsystem2/Action
  If Action Subsystem4/1(Out1) -> Merge1/6
  From Workspace2/1 -> If1/1
  If Action Subsystem6/1(Out1) -> Merge1/5
  Merge1/1 -> Out1/1
  If1/8 -> If Action Subsystem1/Action
  If Action Subsystem3/1(Out1) -> Merge1/7
  In1/1 -> If Action Subsystem1/1(In1), If Action Subsystem3/1(In1), If Action Subsystem4/1(In1), If Action Subsystem7/1(In1), If Action Subsystem8/1(In1), If Action Subsystem9/1(In1), If Action Subsystem5/1(In1), If Action Subsystem6/1(In1), If Action Subsystem10/1(In1), If Action Subsystem2/1(In1)
  If1/6 -> If Action Subsystem4/Action
  If Action Subsystem1/1(Out1) -> Merge1/8
  If1/4 -> If Action Subsystem5/Action
  If Action Subsystem8/1(Out1) -> Merge1/2
  If1/5 -> If Action Subsystem6/Action
  If Action Subsystem7/1(Out1) -> Merge1/3
  If1/3 -> If Action Subsystem7/Action
  If1/7 -> If Action Subsystem3/Action
  If Action Subsystem5/1(Out1) -> Merge1/4
  If Action Subsystem2/1(Out1) -> Merge1/10
  If1/2 -> If Action Subsystem8/Action
  If1/1 -> If Action Subsystem9/Action
  If Action Subsystem9/1(Out1) -> Merge1/1
  If1/9 -> If Action Subsystem10/Action
  If Action Subsystem10/1(Out1) -> Merge1/9

== system LUT_kidney_35/If Action Subsystem6/If Action Subsystem3/If Action Subsystem8 ==
  note: 0.8-0.89
  In1 : Inport
  Action Port : ActionPort  ActionPortLabel=elseif(u1 >= 0.795)
  From Workspace2 : FromWorkspace  VariableName=SimInputHR  Interpolate=off  OutputAfterFinalValue=Setting to zero
  If Action Subsystem1 : Subsystem  TreatAsAtomicUnit=on
  If Action Subsystem10 : Subsystem  TreatAsAtomicUnit=on
  If Action Subsystem2 : Subsystem  TreatAsAtomicUnit=on
  If Action Subsystem3 : Subsystem  TreatAsAtomicUnit=on
  If Action Subsystem4 : Subsystem  TreatAsAtomicUnit=on
  If Action Subsystem5 : Subsystem  TreatAsAtomicUnit=on
  If Action Subsystem6 : Subsystem  TreatAsAtomicUnit=on
  If Action Subsystem7 : Subsystem  TreatAsAtomicUnit=on
  If Action Subsystem8 : Subsystem  TreatAsAtomicUnit=on
  If Action Subsystem9 : Subsystem  TreatAsAtomicUnit=on
  If1 : If  IfExpression=u1 >= 0.885  ElseIfExpressions=u1 >= 0.875, u1 >= 0.865, u1 >= 0.855, u1 >= 0.845, u1 >= 0.835, u1 >= 0.825, u1 >= 0.815, u1 >= 0.805
  Merge1 : Merge  Inputs=10
  Out1 : Outport
  wires:
  If1/10 -> If Action Subsystem2/Action
  If Action Subsystem4/1(Out1) -> Merge1/6
  From Workspace2/1 -> If1/1
  If Action Subsystem6/1(Out1) -> Merge1/5
  Merge1/1 -> Out1/1
  If1/8 -> If Action Subsystem1/Action
  If Action Subsystem3/1(Out1) -> Merge1/7
  In1/1 -> If Action Subsystem1/1(In1), If Action Subsystem3/1(In1), If Action Subsystem4/1(In1), If Action Subsystem7/1(In1), If Action Subsystem8/1(In1), If Action Subsystem9/1(In1), If Action Subsystem5/1(In1), If Action Subsystem6/1(In1), If Action Subsystem10/1(In1), If Action Subsystem2/1(In1)
  If1/6 -> If Action Subsystem4/Action
  If Action Subsystem1/1(Out1) -> Merge1/8
  If1/4 -> If Action Subsystem5/Action
  If Action Subsystem8/1(Out1) -> Merge1/2
  If1/5 -> If Action Subsystem6/Action
  If Action Subsystem7/1(Out1) -> Merge1/3
  If1/3 -> If Action Subsystem7/Action
  If1/7 -> If Action Subsystem3/Action
  If Action Subsystem5/1(Out1) -> Merge1/4
  If Action Subsystem2/1(Out1) -> Merge1/10
  If1/2 -> If Action Subsystem8/Action
  If1/1 -> If Action Subsystem9/Action
  If Action Subsystem9/1(Out1) -> Merge1/1
  If1/9 -> If Action Subsystem10/Action
  If Action Subsystem10/1(Out1) -> Merge1/9

== system LUT_kidney_35/If Action Subsystem6/If Action Subsystem3/If Action Subsystem9 ==
  note: 0.9-0.99
  In2 : Inport
  Action Port : ActionPort  ActionPortLabel=if(u1 >= 0.895)
  From Workspace2 : FromWorkspace  VariableName=SimInputHR  Interpolate=off  OutputAfterFinalValue=Setting to zero
  If Action Subsystem1 : Subsystem  TreatAsAtomicUnit=on
  If Action Subsystem10 : Subsystem  TreatAsAtomicUnit=on
  If Action Subsystem2 : Subsystem  TreatAsAtomicUnit=on
  If Action Subsystem3 : Subsystem  TreatAsAtomicUnit=on
  If Action Subsystem4 : Subsystem  TreatAsAtomicUnit=on
  If Action Subsystem5 : Subsystem  TreatAsAtomicUnit=on
  If Action Subsystem6 : Subsystem  TreatAsAtomicUnit=on
  If Action Subsystem7 : Subsystem  TreatAsAtomicUnit=on
  If Action Subsystem8 : Subsystem  TreatAsAtomicUnit=on
  If Action Subsystem9 : Subsystem  TreatAsAtomicUnit=on
  If1 : If  IfExpression=u1 >= 0.985  ElseIfExpressions=u1 >= 0.975, u1 >= 0.965, u1 >= 0.955, u1 >= 0.945, u1 >= 0.935, u1 >= 0.925, u1 >= 0.915, u1 >= 0.905
  Merge1 : Merge  Inputs=10
  Out2 : Outport
  wires:
  If1/10 -> If Action Subsystem2/Action
  If Action Subsystem4/1(Out1) -> Merge1/6
  From Workspace2/1 -> If1/1
  If Action Subsystem6/1(Out1) -> Merge1/5
  Merge1/1 -> Out2/1
  If1/8 -> If Action Subsystem1/Action
  If Action Subsystem3/1(Out1) -> Merge1/7
  In2/1 -> If Action Subsystem10/1(In1), If Action Subsystem1/1(In1), If Action Subsystem3/1(In1), If Action Subsystem4/1(In1), If Action Subsystem7/1(In1), If Action Subsystem8/1(In1), If Action Subsystem9/1(In1), If Action Subsystem5/1(In1), If Action Subsystem6/1(In1), If Action Subsystem2/1(In1)
  If1/6 -> If Action Subsystem4/Action
  If Action Subsystem1/1(Out1) -> Merge1/8
  If1/4 -> If Action Subsystem5/Action
  If Action Subsystem8/1(Out1) -> Merge1/2
  If1/5 -> If Action Subsystem6/Action
  If Action Subsystem7/1(Out1) -> Merge1/3
  If1/3 -> If Action Subsystem7/Action
  If1/7 -> If Action Subsystem3/Action
  If Action Subsystem5/1(Out1) -> Merge1/4
  If Action Subsystem2/1(Out1) -> Merge1/10
  If1/2 -> If Action Subsystem8/Action
  If1/1 -> If Action Subsystem9/Action
  If Action Subsystem9/1(Out1) -> Merge1/1
  If1/9 -> If Action Subsystem10/Action
  If Action Subsystem10/1(Out1) -> Merge1/9

== system LUT_kidney_35/If Action Subsystem6/If Action Subsystem1/If Action Subsystem5/If Action Subsystem1 ==
  In1 : Inport
  Action Port : ActionPort  ActionPortLabel=elseif( u1 >= 1.115)
  LUT 1.12RR : Lookup_n-D  NumberOfTableDimensions=1  BreakpointsForDimension1=[418.0995;530.6897;621.0357;717.6875;814.4601;911.1126;1007.644;1104.076;1200.433;1296.731;1392.982;1489.196;1585.381;1681.541;1777.681;1873.804;1969.911]  Table=[400;500;600;700;800;900;1000;1100;1200;1300;1400;1500;1600;1700;1800;1900;2000]  InternalRulePriority=Speed  RndMeth=Simplest
  Out1 : Outport
  wires:
  In1/1 -> LUT 1.12RR/1
  LUT 1.12RR/1 -> Out1/1

== system LUT_kidney_35/If Action Subsystem6/If Action Subsystem1/If Action Subsystem5/If Action Subsystem10 ==
  In1 : Inport
  Action Port : ActionPort  ActionPortLabel=elseif( u1 >= 1.105)
  LUT 1.11RR : Lookup_n-D  NumberOfTableDimensions=1  BreakpointsForDimension1=[418.3264;531.0464;621.5073;718.3016;815.2273;912.0394;1008.734;1105.334;1201.861;1298.329;1394.753;1491.141;1587.501;1683.836;1780.152;1876.45;1972.734]  Table=[400;500;600;700;800;900;1000;1100;1200;1300;1400;1500;1600;1700;1800;1900;2000]  InternalRulePriority=Speed  RndMeth=Simplest
  Out1 : Outport
  wires:
  In1/1 -> LUT 1.11RR/1
  LUT 1.11RR/1 -> Out1/1

== system LUT_kidney_35/If Action Subsystem6/If Action Subsystem1/If Action Subsystem5/If Action Subsystem2 ==
  In1 : Inport
  Action Port : ActionPort  ActionPortLabel=else
  LUT 1.10RR : Lookup_n-D  NumberOfTableDimensions=1  BreakpointsForDimension1=[418.5571;531.4108;621.9901;718.9306;816.013;912.9885;1009.851;1106.622;1203.322;1299.966;1396.566;1493.131;1589.669;1686.183;1782.678;1879.157;1975.621]  Table=[400;500;600;700;800;900;1000;1100;1200;1300;1400;1500;1600;1700;1800;1900;2000]  InternalRulePriority=Speed  RndMeth=Simplest
  Out1 : Outport
  wires:
  In1/1 -> LUT 1.10RR/1
  LUT 1.10RR/1 -> Out1/1

== system LUT_kidney_35/If Action Subsystem6/If Action Subsystem1/If Action Subsystem5/If Action Subsystem3 ==
  In1 : Inport
  Action Port : ActionPort  ActionPortLabel=elseif( u1 >= 1.125)
  LUT 1.13RR : Lookup_n-D  NumberOfTableDimensions=1  BreakpointsForDimension1=[417.8761;530.3407;620.5749;717.0878;813.7111;910.2076;1006.578;1102.847;1199.038;1295.168;1391.25;1487.294;1583.308;1679.296;1775.264;1871.214;1967.149]  Table=[400;500;600;700;800;900;1000;1100;1200;1300;1400;1500;1600;1700;1800;1900;2000]  InternalRulePriority=Speed  RndMeth=Simplest
  Out1 : Outport
  wires:
  In1/1 -> LUT 1.13RR/1
  LUT 1.13RR/1 -> Out1/1

== system LUT_kidney_35/If Action Subsystem6/If Action Subsystem1/If Action Subsystem5/If Action Subsystem4 ==
  In1 : Inport
  Action Port : ActionPort  ActionPortLabel=elseif( u1 >= 1.135)
  LUT 1.14RR : Lookup_n-D  NumberOfTableDimensions=1  BreakpointsForDimension1=[417.6561;529.9989;620.1246;716.502;812.9795;909.3235;1005.537;1101.646;1197.674;1293.64;1389.556;1485.434;1581.28;1677.101;1772.9;1868.681;1964.446]  Table=[400;500;600;700;800;900;1000;1100;1200;1300;1400;1500;1600;1700;1800;1900;2000]  InternalRulePriority=Speed  RndMeth=Simplest
  Out1 : Outport
  wires:
  In1/1 -> LUT 1.14RR/1
  LUT 1.14RR/1 -> Out1/1

== system LUT_kidney_35/If Action Subsystem6/If Action Subsystem1/If Action Subsystem5/If Action Subsystem5 ==
  In1 : Inport
  Action Port : ActionPort  ActionPortLabel=elseif( u1 >= 1.155)
  LUT 1.16RR : Lookup_n-D  NumberOfTableDimensions=1  BreakpointsForDimension1=[417.2261;529.3364;619.2539;715.3706;811.5665;907.6159;1003.526;1099.325;1195.038;1290.685;1386.281;1481.835;1577.357;1672.851;1768.323;1863.776;1959.212]  Table=[400;500;600;700;800;900;1000;1100;1200;1300;1400;1500;1600;1700;1800;1900;2000]  InternalRulePriority=Speed  RndMeth=Simplest
  Out1 : Outport
  wires:
  In1/1 -> LUT 1.16RR/1
  LUT 1.16RR/1 -> Out1/1

== system LUT_kidney_35/If Action Subsystem6/If Action Subsystem1/If Action Subsystem5/If Action Subsystem6 ==
  In1 : Inport
  Action Port : ActionPort  ActionPortLabel=elseif( u1 >= 1.145)
  LUT 1.15RR : Lookup_n-D  NumberOfTableDimensions=1  BreakpointsForDimension1=[417.4395;529.6642;619.6843;715.9298;812.2648;908.4599;1004.52;1100.472;1196.341;1292.146;1387.9;1483.615;1579.297;1674.953;1770.587;1866.202;1961.801]  Table=[400;500;600;700;800;900;1000;1100;1200;1300;1400;1500;1600;1700;1800;1900;2000]  InternalRulePriority=Speed  RndMeth=Simplest
  Out1 : Outport
  wires:
  In1/1 -> LUT 1.15RR/1
  LUT 1.15RR/1 -> Out1/1

== system LUT_kidney_35/If Action Subsystem6/If Action Subsystem1/If Action Subsystem5/If Action Subsystem7 ==
  In1 : Inport
  Action Port : ActionPort  ActionPortLabel=elseif( u1 >= 1.165)
  LUT 1.17RR : Lookup_n-D  NumberOfTableDimensions=1  BreakpointsForDimension1=[417.0159;529.0152;618.8329;714.8241;810.8842;906.7911;1002.554;1098.203;1193.763;1289.256;1384.696;1480.094;1575.458;1670.794;1766.107;1861.4;1956.677]  Table=[400;500;600;700;800;900;1000;1100;1200;1300;1400;1500;1600;1700;1800;1900;2000]  InternalRulePriority=Speed  RndMeth=Simplest
  Out1 : Outport
  wires:
  In1/1 -> LUT 1.17RR/1
  LUT 1.17RR/1 -> Out1/1

== system LUT_kidney_35/If Action Subsystem6/If Action Subsystem1/If Action Subsystem5/If Action Subsystem8 ==
  In1 : Inport
  Action Port : ActionPort  ActionPortLabel=elseif(u1 >= 1.175)
  LUT 1.18RR : Lookup_n-D  NumberOfTableDimensions=1  BreakpointsForDimension1=[416.8086;528.7004;618.4211;714.2899;810.2173;905.9849;1001.604;1097.105;1192.517;1287.858;1383.146;1478.39;1573.599;1668.78;1763.937;1859.075;1954.195]  Table=[400;500;600;700;800;900;1000;1100;1200;1300;1400;1500;1600;1700;1800;1900;2000]  InternalRulePriority=Speed  RndMeth=Simplest
  Out1 : Outport
  wires:
  In1/1 -> LUT 1.18RR/1
  LUT 1.18RR/1 -> Out1/1

== system LUT_kidney_35/If Action Subsystem6/If Action Subsystem1/If Action Subsystem5/If Action Subsystem9 ==
  In1 : Inport
  Action Port : ActionPort  ActionPortLabel=if(u1 >= 1.185)
  LUT 1.19RR : Lookup_n-D  NumberOfTableDimensions=1  BreakpointsForDimension1=[416.6044;528.3919;618.0181;713.7676;809.5654;905.1967;1000.675;1096.032;1191.297;1286.491;1381.628;1476.722;1571.78;1666.808;1761.813;1856.797;1951.764]  Table=[400;500;600;700;800;900;1000;1100;1200;1300;1400;1500;1600;1700;1800;1900;2000]  InternalRulePriority=Speed  RndMeth=Simplest
  Out1 : Outport
  wires:
  In1/1 -> LUT 1.19RR/1
  LUT 1.19RR/1 -> Out1/1

== system LUT_kidney_35/If Action Subsystem6/If Action Subsystem1/If Action Subsystem6/If Action Subsystem1 ==
  In1 : Inport
  Action Port : ActionPort  ActionPortLabel=elseif( u1 >= 1.015)
  LUT 1.02RR : Lookup_n-D  NumberOfTableDimensions=1  BreakpointsForDimension1=[420.5519;534.646;626.3059;724.5665;823.0539;921.4868;1019.842;1118.131;1216.366;1314.559;1412.719;1510.852;1608.964;1707.058;1805.137;1903.203;2001.256]  Table=[400;500;600;700;800;900;1000;1100;1200;1300;1400;1500;1600;1700;1800;1900;2000]  InternalRulePriority=Speed  RndMeth=Simplest
  Out1 : Outport
  wires:
  In1/1 -> LUT 1.02RR/1
  LUT 1.02RR/1 -> Out1/1

== system LUT_kidney_35/If Action Subsystem6/If Action Subsystem1/If Action Subsystem6/If Action Subsystem10 ==
  In1 : Inport
  Action Port : ActionPort  ActionPortLabel=elseif( u1 >= 1.005)
  LUT 1.01RR : Lookup_n-D  NumberOfTableDimensions=1  BreakpointsForDimension1=[420.8224;535.0958;626.9096;725.3562;824.0403;922.6765;1021.239;1119.739;1218.186;1316.594;1414.969;1513.32;1611.649;1709.961;1808.259;1906.545;2004.817]  Table=[400;500;600;700;800;900;1000;1100;1200;1300;1400;1500;1600;1700;1800;1900;2000]  InternalRulePriority=Speed  RndMeth=Simplest
  Out1 : Outport
  wires:
  In1/1 -> LUT 1.01RR/1
  LUT 1.01RR/1 -> Out1/1

== system LUT_kidney_35/If Action Subsystem6/If Action Subsystem1/If Action Subsystem6/If Action Subsystem2 ==
  In1 : Inport
  Action Port : ActionPort  ActionPortLabel=else
  LUT 1.00RR : Lookup_n-D  NumberOfTableDimensions=1  BreakpointsForDimension1=[421.0983;535.557;627.5295;726.1674;825.0535;923.898;1022.674;1121.389;1220.054;1318.682;1417.278;1515.85;1614.402;1712.938;1811.46;1909.97;2008.467]  Table=[400;500;600;700;800;900;1000;1100;1200;1300;1400;1500;1600;1700;1800;1900;2000]  InternalRulePriority=Speed  RndMeth=Simplest
  Out1 : Outport
  wires:
  In1/1 -> LUT 1.00RR/1
  LUT 1.00RR/1 -> Out1/1

== system LUT_kidney_35/If Action Subsystem6/If Action Subsystem1/If Action Subsystem6/If Action Subsystem3 ==
  In1 : Inport
  Action Port : ActionPort  ActionPortLabel=elseif( u1 >= 1.025)
  LUT 1.03RR : Lookup_n-D  NumberOfTableDimensions=1  BreakpointsForDimension1=[420.2865;534.2073;625.7178;723.7974;822.0932;920.3279;1018.481;1116.564;1214.591;1312.575;1410.524;1508.445;1606.345;1704.225;1802.091;1899.942;1997.781]  Table=[400;500;600;700;800;900;1000;1100;1200;1300;1400;1500;1600;1700;1800;1900;2000]  InternalRulePriority=Speed  RndMeth=Simplest
  Out1 : Outport
  wires:
  In1/1 -> LUT 1.03RR/1
  LUT 1.03RR/1 -> Out1/1
